simulink model "Amf"  (Simulink 8.4)
settings: Solver=ode45  StartTime=0.0  StopTime=10.0  RelTol=1e-3
undefined symbols (not defined in the file): Amf_facRelAirMan, Amf_flgAirMassPerStrOverride, Amf_flgRelAirOverride, Amf_flgSwitch2AirMassFlowMeter, Amf_mAirPerStrMan, Amf_shcSpecGasConst_C, Amf_volEngDisp_C
settings Model: Creator=YAL9FE  LastModifiedBy=ric9fe
settings DebuggingCC: FcnCallInpInsideContextMsg=EnableAllAsWarning

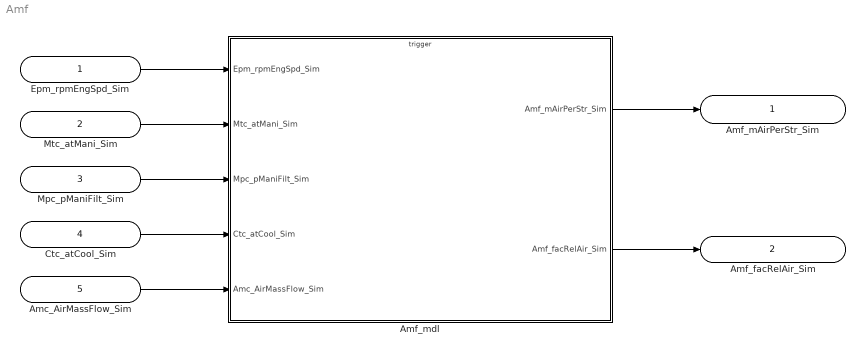
== system Amf ==
  Epm_rpmEngSpd_Sim : Inport
  Mtc_atMani_Sim : Inport  Port=2
  Mpc_pManiFilt_Sim : Inport  Port=3
  Ctc_atCool_Sim : Inport  Port=4
  Amc_AirMassFlow_Sim : Inport  Port=5
  Amf_mdl : Subsystem  mask(Functions){}
      mask help: AirMassFlow
      mask Display:
      | image(imread('AirMassFlow.jpg'))
      | port_label('input',1,'Epm_rpmEngSpd_Sim')
      | port_label('input',2,'Mtc_atMani_Sim')
      | port_label('input',3,'Mpc_pManiFilt_Sim')
      | port_label('input',4,'Ctc_atCool_Sim')
      | port_label('input',5,'Amc_AirMassFlow_Sim')
      | port_label('output',1,'Amf_mAirPerStr_Sim')
      | port_label('output',2,'Amf_facRelAir_Sim')
  Amf_mAirPerStr_Sim : Outport
  Amf_facRelAir_Sim : Outport  Port=2
  wires:
  Epm_rpmEngSpd_Sim/1 -> Amf_mdl/1(Epm_rpmEngSpd_Sim)
  Mtc_atMani_Sim/1 -> Amf_mdl/2(Mtc_atMani_Sim)
  Mpc_pManiFilt_Sim/1 -> Amf_mdl/3(Mpc_pManiFilt_Sim)
  Ctc_atCool_Sim/1 -> Amf_mdl/4(Ctc_atCool_Sim)
  Amc_AirMassFlow_Sim/1 -> Amf_mdl/5(Amc_AirMassFlow_Sim)
  Amf_mdl/1(Amf_mAirPerStr_Sim) -> Amf_mAirPerStr_Sim/1
  Amf_mdl/2(Amf_facRelAir_Sim) -> Amf_facRelAir_Sim/1

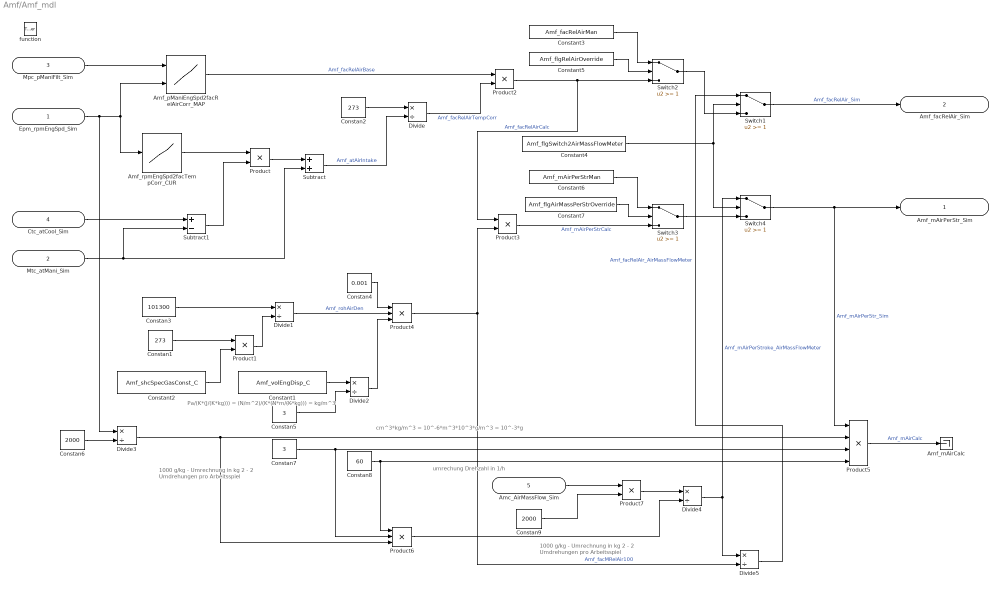
== system Amf/Amf_mdl ==
  note: Pa/(K*(J/(K*kg))) = (N/m^2)/(K*(N*m/(K*kg))) = kg/m^3
  note: cm^3*kg/m^3 = 10^-6*m^3*10^3*g/m^3 = 10^-3*g
  note: 1000 g/kg - Umrechnung in kg
      | 2 - 2 Umdrehungen pro Arbeitsspiel
  note: umrechung Drehzahl in 1/h
  note: 1000 g/kg - Umrechnung in kg
      | 2 - 2 Umdrehungen pro Arbeitsspiel
  Epm_rpmEngSpd_Sim : Inport
  Mtc_atMani_Sim : Inport  Port=2
  Mpc_pManiFilt_Sim : Inport  Port=3
  Ctc_atCool_Sim : Inport  Port=4
  Amc_AirMassFlow_Sim : Inport  Port=5
  function : TriggerPort  TriggerType=function-call
  Amf_mAirCalc : Terminator
  Amf_pManiEngSpd2facRelAirCorr_MAP : Lookup_n-D  BreakpointsForDimension1=[1:3]  BreakpointsForDimension2=[1:3]  ExtrapMethod=Clip  InputSameDT=on
  Amf_rpmEngSpd2facTempCorr_CUR : Lookup_n-D  NumberOfTableDimensions=1  BreakpointsForDimension1=[1:3]  Table=[1 2 3]  ExtrapMethod=Clip  InputSameDT=on
  Constan1 : Constant  Value=273  OutDataTypeStr=single
  Constan2 : Constant  Value=273  OutDataTypeStr=single
  Constan3 : Constant  Value=101300  OutDataTypeStr=single
  Constan4 : Constant  Value=0.001  OutMin=0  OutDataTypeStr=single
  Constan5 : Constant  Value=3  OutDataTypeStr=single
  Constan6 : Constant  Value=2000  OutDataTypeStr=single
  Constan7 : Constant  Value=3  OutDataTypeStr=single
  Constan8 : Constant  Value=60  OutDataTypeStr=single
  Constan9 : Constant  Value=2000  OutDataTypeStr=single
  Constant1 : Constant  Value=Amf_volEngDisp_C
  Constant2 : Constant  Value=Amf_shcSpecGasConst_C
  Constant3 : Constant  Value=Amf_facRelAirMan
  Constant4 : Constant  Value=Amf_flgSwitch2AirMassFlowMeter
  Constant5 : Constant  Value=Amf_flgRelAirOverride
  Constant6 : Constant  Value=Amf_mAirPerStrMan
  Constant7 : Constant  Value=Amf_flgAirMassPerStrOverride
  Divide{,1..5} (6 alike) : Product  Inputs=*/  OutDataTypeStr=Inherit: Same as first input
  Product{,1..3,7} (5 alike) : Product  OutDataTypeStr=Inherit: Same as first input
  Product4 : Product  Inputs=3  OutDataTypeStr=Inherit: Same as first input
  Product5 : Product  Inputs=4  OutDataTypeStr=Inherit: Same as first input
  Product6 : Product  Inputs=3  OutDataTypeStr=Inherit: Same as first input
  Subtract : Sum  OutDataTypeStr=Inherit: Same as first input
  Subtract1 : Sum  Inputs=+-  OutDataTypeStr=Inherit: Same as first input
  Switch{1..4} (4 alike) : Switch  Threshold=1
  Amf_mAirPerStr_Sim : Outport
  Amf_facRelAir_Sim : Outport  Port=2
  wires:
  Epm_rpmEngSpd_Sim/1 -> Amf_pManiEngSpd2facRelAirCorr_MAP/2, Amf_rpmEngSpd2facTempCorr_CUR/1, Divide3/1
  Mpc_pManiFilt_Sim/1 -> Amf_pManiEngSpd2facRelAirCorr_MAP/1
  Amf_rpmEngSpd2facTempCorr_CUR/1 -> Product/1
  Product/1 -> Subtract/1
  Ctc_atCool_Sim/1 -> Subtract1/1
  Mtc_atMani_Sim/1 -> Subtract1/2, Subtract/2
  Subtract1/1 -> Product/2
  Constan2/1 -> Divide/1
  Subtract/1 -> Divide/2  "Amf_atAirIntake"
  Constan3/1 -> Divide1/1
  Constan1/1 -> Product1/1
  Product1/1 -> Divide1/2
  Constant2/1 -> Product1/2
  Divide/1 -> Product2/2  "Amf_facRelAirTempCorr"
  Amf_pManiEngSpd2facRelAirCorr_MAP/1 -> Product2/1  "Amf_facRelAirBase"
  Divide1/1 -> Product4/2  "Amf_rohAirDen"
  Constant1/1 -> Divide2/1
  Constan5/1 -> Divide2/2
  Constan4/1 -> Product4/1
  Divide2/1 -> Product4/3
  Product2/1 -> Product3/1, Switch2/3  "Amf_facRelAirCalc"
  Product4/1 -> Product3/2, Divide5/2  "Amf_facMRelAir100"
  Switch2/1 -> Switch1/3
  Constant5/1 -> Switch2/2
  Constant3/1 -> Switch2/1
  Switch1/1 -> Amf_facRelAir_Sim/1  "Amf_facRelAir_Sim"
  Constant4/1 -> Switch4/2, Switch1/2
  Constant7/1 -> Switch3/2
  Constant6/1 -> Switch3/1
  Product3/1 -> Switch3/3  "Amf_mAirPerStrCalc"
  Switch3/1 -> Switch4/3
  Switch4/1 -> Amf_mAirPerStr_Sim/1, Product5/1  "Amf_mAirPerStr_Sim"
  Constan6/1 -> Divide3/2
  Product5/1 -> Amf_mAirCalc/1  "Amf_mAirCalc"
  Divide3/1 -> Product5/2, Product6/3
  Constan7/1 -> Product5/3, Product6/2
  Constan8/1 -> Product5/4, Product6/1
  Amc_AirMassFlow_Sim/1 -> Product7/1
  Constan9/1 -> Product7/2
  Product7/1 -> Divide4/1
  Product6/1 -> Divide4/2
  Divide4/1 -> Divide5/1, Switch4/1  "Amf_mAirPerStroke_AirMassFlowMeter"
  Divide5/1 -> Switch1/1  "Amf_facRelAir_AirMassFlowMeter"
